simulink model "acvh_controller_mark1"  (R2020b)
settings: Solver=FixedStepAuto  StartTime=0.0  StopTime=Inf  RelTol=1e-3  EnableMultiTasking=on
values from neighbouring files (symbols this model uses):
  D = .2540    (= 0.254)    [iris_quadcopter_specs.m]
  SampleTime = 0.001    [iris_quadcopter_specs.m]
undefined symbols (not defined in the file or in its folder): dev, DiscIntNeverNeededParam, Main, pwm_output0
libraries: pid_lib x6, px4uORBlib x5, sharedtransform x1, px4lib x1
settings Model: SimulationMode=external  ExtModeTrigDuration=10  Creator=sid  LastModifiedBy=sid
settings SolverCC: PositivePriorityOrder=on
settings OptimizationCC: EnhancedBackFolding=on  PassReuseOutputArgsAs=Individual arguments  ZeroExternalMemoryAtStartup=off  ZeroInternalMemoryAtStartup=off  MaxStackSize=64  OptimizeBlockOrder=speed  DifferentSizesBufferReuse=on  OptimizationCustomize=off  EfficientTunableParamExpr=on
settings DebuggingCC: ParameterTunabilityLossMsg=error
settings HardwareCC: ProdBitPerPointer=32  ProdBitPerSizeT=32  ProdBitPerPtrDiffT=32  ProdLargestAtomicInteger=Long  ProdLargestAtomicFloat=Double  ProdWordSize=32  ProdLongLongMode=on  ProdHWDeviceType=ARM Compatible->ARM Cortex
settings SFSimCC: MATLABDynamicMemAlloc=off  SimTargetLang=C++
settings RTWCC: Description=Embedded Coder  SystemTargetFile=ert.tlc  HardwareBoard=PX4 Host Target  TLCOptions="-aInlineSetEventsForThisBaseRateFcn=TLC_FALSE -aSuppressMultiTaskScheduler=TLC_FALSE  -aRateBasedStepFcn=0"  TemplateMakefile=ert_default_tmf  Toolchain=GNU Tools for PX4 Autopilots  PortableWordSizes=on  TargetLang=C++
settings CodeAppCC: ForceParamTrailComments=on  IgnoreCustomStorageClasses=off  OperatorAnnotations=on  SimulinkDataObjDesc=on  SFDataObjDesc=on  InsertBlockDesc=on
settings ERTTargetCC: ExtMode=on  ExtModeMexArgs='127.0.0.1' 1 17725

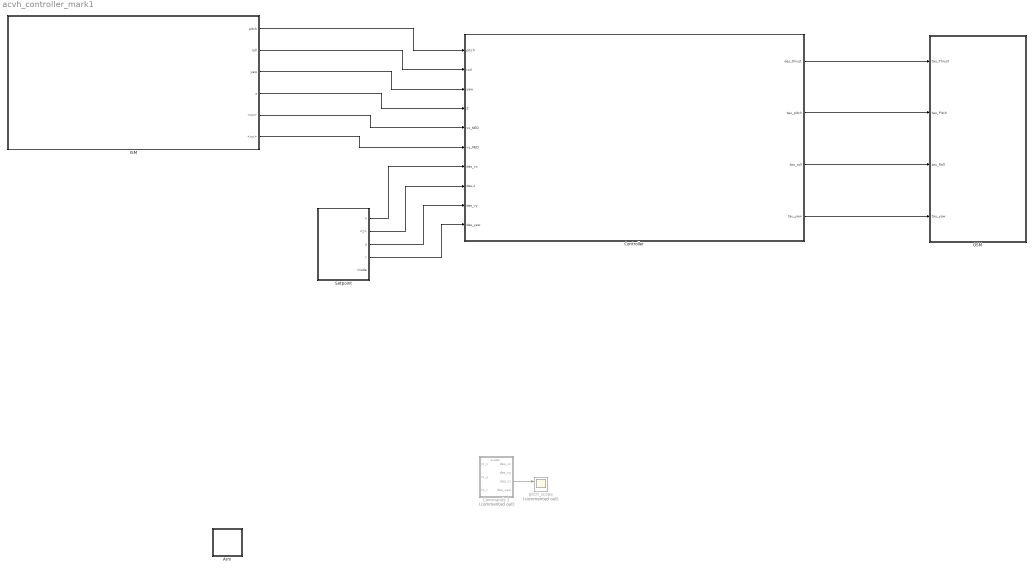
== system acvh_controller_mark1 ==
  Arm : Subsystem
  Commands 1 : Subsystem  Commented=on
  Controller : Subsystem
  ISM : Subsystem
  OSM : Subsystem
  Setpoint : Subsystem
  pitch_scope : Scope  Commented=on  NumInputPorts=2
  wires:
  Controller/1(des_thrust) -> OSM/1(tau_Thrust)
  Controller/3(tau_roll) -> OSM/3(tau_Roll)
  Controller/4(tau_yaw) -> OSM/4(tau_yaw)
  Commands 1/3(des_vz) -> pitch_scope/1
  Controller/2(tau_pitch) -> OSM/2(tau_Pitch)
  ISM/1(pitch) -> Controller/1(pitch)
  ISM/2(roll) -> Controller/2(roll)
  ISM/3(yaw) -> Controller/3(yaw)
  ISM/4(z) -> Controller/4(Z)
  ISM/5(<vx>) -> Controller/5(vx_NED)
  ISM/6(<vy>) -> Controller/6(vy_NED)
  Setpoint/4(r) -> Controller/10(des_yaw)
  Setpoint/1(x) -> Controller/7(des_vx)
  Setpoint/3(y) -> Controller/9(des_vy)
  Setpoint/2(<z>) -> Controller/8(des-z)

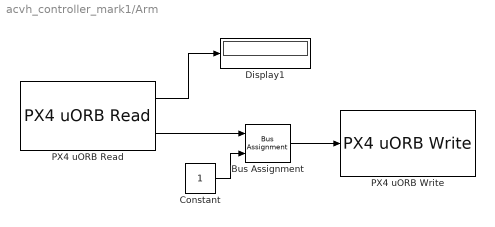
== system acvh_controller_mark1/Arm ==
  Bus Assignment : BusAssignment  AssignedSignals=armed
  Constant : Constant  OutDataTypeStr=Inherit: Inherit via back propagation  SampleTime=SampleTime
  Display1 : Display
  PX4 uORB Read : px4uORBlib/PX4 uORB Read  uORBTopic=actuator_armed  selectInstance=actuator_armed  SampleTime=SampleTime  BlockingMode=off  BlockTimeout=1e-3
      settings: SourceProductBaseCode=PX4AUTOPILOTS
  PX4 uORB Write : px4uORBlib/PX4 uORB Write  uORBTopic=actuator_armed  selectInstance=actuator_armed  MessageQueueLen=1
      settings: SourceProductBaseCode=PX4AUTOPILOTS
  wires:
  PX4 uORB Read/2 -> Bus Assignment/1
  PX4 uORB Read/1 -> Display1/1
  Bus Assignment/1 -> PX4 uORB Write/1
  Constant/1 -> Bus Assignment/2

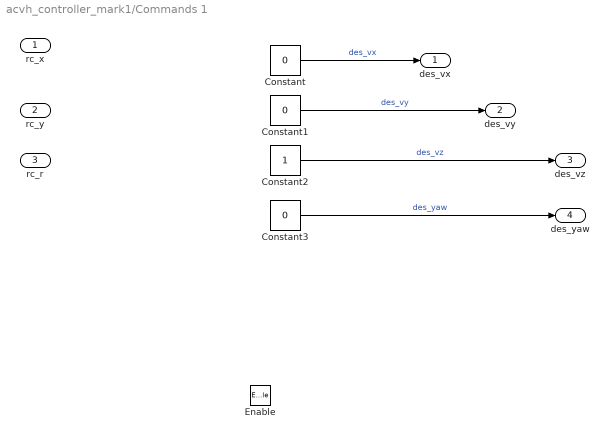
== system acvh_controller_mark1/Commands 1 ==
  rc_x : Inport
  rc_y : Inport  Port=2
  rc_r : Inport  Port=3
  Enable : EnablePort
  Constant : Constant  Value=0
  Constant1 : Constant  Value=0
  Constant2 : Constant
  Constant3 : Constant  Value=0
  des_vx : Outport
  des_vy : Outport  Port=2
  des_vz : Outport  Port=3
  des_yaw : Outport  Port=4
  wires:
  Constant1/1 -> des_vy/1  "des_vy"
  Constant/1 -> des_vx/1  "des_vx"
  Constant2/1 -> des_vz/1  "des_vz"
  Constant3/1 -> des_yaw/1  "des_yaw"

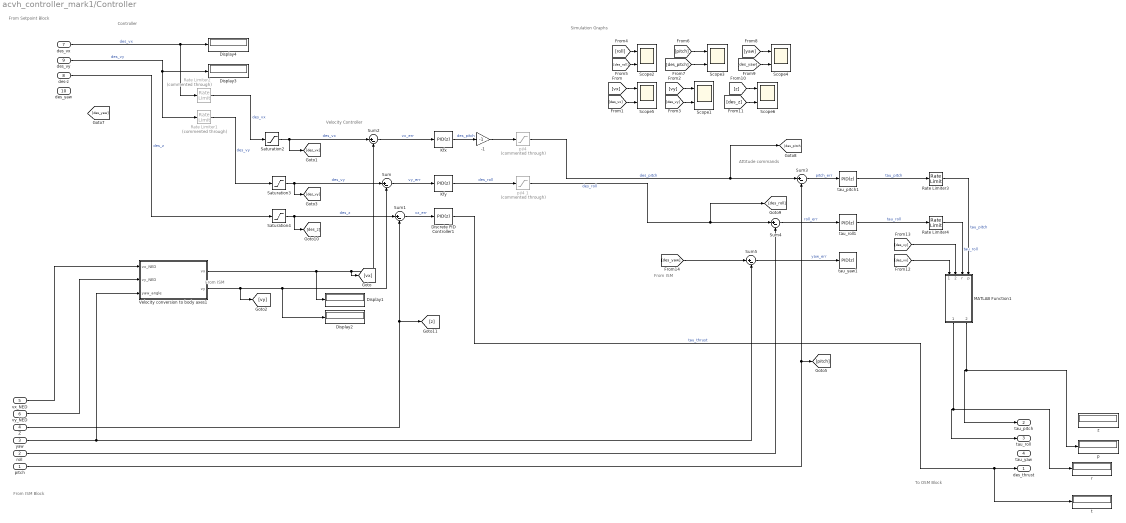
== system acvh_controller_mark1/Controller ==
  note: Simulation Graphs
  note: From Setpoint Block
  note: From ISM
  note: From ISM
  note: Controller
  note: Attitude commands
  note: Velocity Controller
  note: From ISM Block
  note: To OSM Block
  pitch : Inport
  roll : Inport  Port=2
  yaw : Inport  Port=3
  Z : Inport  Port=4
  vx_NED : Inport  Port=5
  vy_NED : Inport  Port=6
  des_vx : Inport  Port=7
  des-z : Inport  Port=8
  des_vy : Inport  Port=9
  des_yaw : Inport  Port=10
  -1 : Gain  Gain=-1
  Discrete PID Controller1 : pid_lib/PID Controller  Controller=PID  Form=Parallel  TimeDomain=Discrete-time  UseExternalTs=off  SampleTime=SampleTime  IntegratorMethod=Trapezoidal  FilterMethod=Trapezoidal  ControllerParametersSource=internal  P=-0.0534535340221691  I=-0.00566953766767209  D=-0.123220888476467  UseFilter=on  N=26.3491959083223  TunerSelectOption=Transfer Function Based (PID Tuner App)  InitialConditionSource=internal  InitialConditionForIntegrator=0  InitialConditionForFilter=0  DifferentiatorICPrevScaledInput=0  ExternalReset=none  TrackingMode=off  Kt=1  LimitOutput=off  SatLimitsSource=internal  UpperSaturationLimit=10  LowerSaturationLimit=-.05  LinearizeAsGain=off  AntiWindupMode=back-calculation  Kb=10  POutMin=[]  POutMax=[]  IOutMin=[]  IOutMax=[]  DOutMin=[]  DOutMax=[]  NOutMin=[]  NOutMax=[]  SumOutMin=[]  SumOutMax=[]  SaturationOutMin=[]  SaturationOutMax=[]  PParamMin=[]  PParamMax=[]  IParamMin=[]  IParamMax=[]  DParamMin=[]  DParamMax=[]  NParamMin=[]  NParamMax=[]  KbParamMin=[]  KbParamMax=[]  KtParamMin=[]  KtParamMax=[]  KbOutMin=[]  KbOutMax=[]  KtOutMin=[]  KtOutMax=[]  IntegratorOutMin=[]  IntegratorOutMax=[]  FilterOutMin=[]  FilterOutMax=[]  SumI1OutMin=[]  SumI1OutMax=[]  SumI2OutMin=[]  SumI2OutMax=[]  SumI3OutMin=[]  SumI3OutMax=[]  SumI4OutMin=[]  SumI4OutMax=[]  SumDOutMin=[]  SumDOutMax=[]  DifferentiatorOutMin=[]  DifferentiatorOutMax=[]  FilterDiffOutCoefMin=[]  FilterDiffOutCoefMax=[]  ReciprocalOutMin=[]  ReciprocalOutMax=[]  SumDenOutMin=[]  SumDenOutMax=[]  SumNumOutMin=[]  SumNumOutMax=[]  DivideOutMin=[]  DivideOutMax=[]  UdiffTsProdOutMin=[]  UdiffTsProdOutMax=[]  NTsProdOutMin=[]  NTsProdOutMax=[]  UintegralTsProdOutMin=[]  UintegralTsProdOutMax=[]  UngainTsProdOutMin=[]  UngainTsProdOutMax=[]  IntegratorContinuousStateAttributes=''  IntegratorStateMustResolveToSignalObject=off  IntegratorRTWStateStorageClass=Auto  FilterContinuousStateAttributes=''  FilterStateMustResolveToSignalObject=off  FilterRTWStateStorageClass=Auto  ParallelPVariant=InternalParameters  IdealPVariant=Disabled  IVariant=InternalParameters  DVariant=InternalParameters  IntegratorVariant=Discrete  SatVariant=Disabled  AWVariant=Passthrough  PCopyVariant=Disabled  TRVariant=Disabled  FdbkBlocksVariant=Forward  IdealPFdbkVariant=Disabled  SatFdbkVariant=Disabled  DerivativeFilterVariant=TrapezoidalFilter  NVariant=InternalParameters  NCopyVariant=InternalParameters  FilterICVariant=InternalICsFilter  IntegratorICVariant=InternalICs  ExternalResetVariant=Disabled  TRSumVariant=Passthrough  SumFdbkVariant=Disabled  SumVariant=Sum_PID  TsampFilterVariant=InternalTs  TsampNgainVariant=Passthrough  TsampIntegralVariant=Passthrough  ExternalSaturationOutDataTypeStr=Inherit: Same as second input
  Display{1..4} (4 alike) : Display
  Kfx : pid_lib/PID Controller  Controller=PID  Form=Parallel  TimeDomain=Discrete-time  UseExternalTs=off  SampleTime=SampleTime  IntegratorMethod=Forward Euler  FilterMethod=Forward Euler  ControllerParametersSource=internal  P=0.183358617742533  I=0.0739424315877928  D=-0.024031657470412  UseFilter=on  N=7.50922781087257  TunerSelectOption=Transfer Function Based (PID Tuner App)  InitialConditionSource=internal  InitialConditionForIntegrator=0  InitialConditionForFilter=0  DifferentiatorICPrevScaledInput=0  ExternalReset=none  TrackingMode=off  Kt=1  LimitOutput=on  SatLimitsSource=internal  UpperSaturationLimit=pi/8  LowerSaturationLimit=-pi/8  LinearizeAsGain=off  AntiWindupMode=clamping  Kb=1  POutMin=[]  POutMax=[]  IOutMin=[]  IOutMax=[]  DOutMin=[]  DOutMax=[]  NOutMin=[]  NOutMax=[]  SumOutMin=[]  SumOutMax=[]  SaturationOutMin=[]  SaturationOutMax=[]  PParamMin=[]  PParamMax=[]  IParamMin=[]  IParamMax=[]  DParamMin=[]  DParamMax=[]  NParamMin=[]  NParamMax=[]  KbParamMin=[]  KbParamMax=[]  KtParamMin=[]  KtParamMax=[]  KbOutMin=[]  KbOutMax=[]  KtOutMin=[]  KtOutMax=[]  IntegratorOutMin=[]  IntegratorOutMax=[]  FilterOutMin=[]  FilterOutMax=[]  SumI1OutMin=[]  SumI1OutMax=[]  SumI2OutMin=[]  SumI2OutMax=[]  SumI3OutMin=[]  SumI3OutMax=[]  SumI4OutMin=[]  SumI4OutMax=[]  SumDOutMin=[]  SumDOutMax=[]  DifferentiatorOutMin=[]  DifferentiatorOutMax=[]  FilterDiffOutCoefMin=[]  FilterDiffOutCoefMax=[]  ReciprocalOutMin=[]  ReciprocalOutMax=[]  SumDenOutMin=[]  SumDenOutMax=[]  SumNumOutMin=[]  SumNumOutMax=[]  DivideOutMin=[]  DivideOutMax=[]  UdiffTsProdOutMin=[]  UdiffTsProdOutMax=[]  NTsProdOutMin=[]  NTsProdOutMax=[]  UintegralTsProdOutMin=[]  UintegralTsProdOutMax=[]  UngainTsProdOutMin=[]  UngainTsProdOutMax=[]  IntegratorContinuousStateAttributes=''  IntegratorStateMustResolveToSignalObject=off  IntegratorRTWStateStorageClass=Auto  FilterContinuousStateAttributes=''  FilterStateMustResolveToSignalObject=off  FilterRTWStateStorageClass=Auto  ParallelPVariant=InternalParameters  IdealPVariant=Disabled  IVariant=InternalParameters  DVariant=InternalParameters  IntegratorVariant=Discrete  SatVariant=Enabled  AWVariant=DiscClampingParallel  PCopyVariant=Disabled  TRVariant=Disabled  FdbkBlocksVariant=Forward  IdealPFdbkVariant=Disabled  SatFdbkVariant=Disabled  DerivativeFilterVariant=ForwardEulerFilter  NVariant=InternalParameters  NCopyVariant=Disabled  FilterICVariant=InternalICsFilter  IntegratorICVariant=InternalICs  ExternalResetVariant=Disabled  TRSumVariant=Passthrough  SumFdbkVariant=Disabled  SumVariant=Sum_PID  TsampFilterVariant=InternalTs  TsampNgainVariant=Passthrough  TsampIntegralVariant=Passthrough  ExternalSaturationOutDataTypeStr=Inherit: Same as second input
  Kfy : pid_lib/PID Controller  Controller=PID  Form=Parallel  TimeDomain=Discrete-time  UseExternalTs=off  SampleTime=SampleTime  IntegratorMethod=Forward Euler  FilterMethod=Forward Euler  ControllerParametersSource=internal  P=0.183358617742446  I=0.0739424315877666  D=-0.0240316574704006  UseFilter=on  N=7.50922781087257  TunerSelectOption=Transfer Function Based (PID Tuner App)  InitialConditionSource=internal  InitialConditionForIntegrator=0  InitialConditionForFilter=0  DifferentiatorICPrevScaledInput=0  ExternalReset=none  TrackingMode=off  Kt=1  LimitOutput=on  SatLimitsSource=internal  UpperSaturationLimit=pi/8  LowerSaturationLimit=-pi/8  LinearizeAsGain=off  AntiWindupMode=clamping  Kb=1  POutMin=[]  POutMax=[]  IOutMin=[]  IOutMax=[]  DOutMin=[]  DOutMax=[]  NOutMin=[]  NOutMax=[]  SumOutMin=[]  SumOutMax=[]  SaturationOutMin=[]  SaturationOutMax=[]  PParamMin=[]  PParamMax=[]  IParamMin=[]  IParamMax=[]  DParamMin=[]  DParamMax=[]  NParamMin=[]  NParamMax=[]  KbParamMin=[]  KbParamMax=[]  KtParamMin=[]  KtParamMax=[]  KbOutMin=[]  KbOutMax=[]  KtOutMin=[]  KtOutMax=[]  IntegratorOutMin=[]  IntegratorOutMax=[]  FilterOutMin=[]  FilterOutMax=[]  SumI1OutMin=[]  SumI1OutMax=[]  SumI2OutMin=[]  SumI2OutMax=[]  SumI3OutMin=[]  SumI3OutMax=[]  SumI4OutMin=[]  SumI4OutMax=[]  SumDOutMin=[]  SumDOutMax=[]  DifferentiatorOutMin=[]  DifferentiatorOutMax=[]  FilterDiffOutCoefMin=[]  FilterDiffOutCoefMax=[]  ReciprocalOutMin=[]  ReciprocalOutMax=[]  SumDenOutMin=[]  SumDenOutMax=[]  SumNumOutMin=[]  SumNumOutMax=[]  DivideOutMin=[]  DivideOutMax=[]  UdiffTsProdOutMin=[]  UdiffTsProdOutMax=[]  NTsProdOutMin=[]  NTsProdOutMax=[]  UintegralTsProdOutMin=[]  UintegralTsProdOutMax=[]  UngainTsProdOutMin=[]  UngainTsProdOutMax=[]  IntegratorContinuousStateAttributes=''  IntegratorStateMustResolveToSignalObject=off  IntegratorRTWStateStorageClass=Auto  FilterContinuousStateAttributes=''  FilterStateMustResolveToSignalObject=off  FilterRTWStateStorageClass=Auto  ParallelPVariant=InternalParameters  IdealPVariant=Disabled  IVariant=InternalParameters  DVariant=InternalParameters  IntegratorVariant=Discrete  SatVariant=Enabled  AWVariant=DiscClampingParallel  PCopyVariant=Disabled  TRVariant=Disabled  FdbkBlocksVariant=Forward  IdealPFdbkVariant=Disabled  SatFdbkVariant=Disabled  DerivativeFilterVariant=ForwardEulerFilter  NVariant=InternalParameters  NCopyVariant=Disabled  FilterICVariant=InternalICsFilter  IntegratorICVariant=InternalICs  ExternalResetVariant=Disabled  TRSumVariant=Passthrough  SumFdbkVariant=Disabled  SumVariant=Sum_PID  TsampFilterVariant=InternalTs  TsampNgainVariant=Passthrough  TsampIntegralVariant=Passthrough  ExternalSaturationOutDataTypeStr=Inherit: Same as second input
  MATLAB Function1 : MATLAB Function  TreatAsAtomicUnit=on
  Rate Limiter1 : RateLimiter  Commented=through  RisingSlewLimit=3  FallingSlewLimit=-3
  Rate Limiter2 : RateLimiter  Commented=through  RisingSlewLimit=3  FallingSlewLimit=-3
  Rate Limiter3 : RateLimiter  RisingSlewLimit=.001  FallingSlewLimit=-.001  SampleTimeMode=inherited
  Rate Limiter4 : RateLimiter  RisingSlewLimit=.001  FallingSlewLimit=-.001  SampleTimeMode=inherited
  Saturation2 : Saturate  UpperLimit=8  LowerLimit=-8  LinearizeAsGain=off
  Saturation3 : Saturate  UpperLimit=8  LowerLimit=-8  LinearizeAsGain=off
  Saturation4 : Saturate  UpperLimit=0  LowerLimit=-6
  Scope{1..6} (6 alike) : Scope  NumInputPorts=2
  Sum{,1..5} (6 alike) : Sum  Inputs=|+-
  Velocity conversion to body axes1 : Subsystem
  p : Display
  pi/4 : Saturate  Commented=through  UpperLimit=pi/16  LowerLimit=-pi/16
  pi/4 1 : Saturate  Commented=through  UpperLimit=pi/16  LowerLimit=-pi/16
  r : Display
  t : Display
  tau_pitch1 : pid_lib/PID Controller  Controller=PID  Form=Parallel  TimeDomain=Discrete-time  UseExternalTs=off  SampleTime=SampleTime  IntegratorMethod=Forward Euler  FilterMethod=Forward Euler  ControllerParametersSource=internal  P=0.0543673511512337  I=0.0109980209644375  D=0.0263229670839572  UseFilter=on  N=347.83750102845  TunerSelectOption=Transfer Function Based (PID Tuner App)  InitialConditionSource=internal  InitialConditionForIntegrator=0  InitialConditionForFilter=0  DifferentiatorICPrevScaledInput=0  ExternalReset=none  TrackingMode=off  Kt=1  LimitOutput=on  SatLimitsSource=internal  UpperSaturationLimit=.0005  LowerSaturationLimit=-.0005  LinearizeAsGain=off  AntiWindupMode=none  Kb=1  POutMin=[]  POutMax=[]  IOutMin=[]  IOutMax=[]  DOutMin=[]  DOutMax=[]  NOutMin=[]  NOutMax=[]  SumOutMin=[]  SumOutMax=[]  SaturationOutMin=[]  SaturationOutMax=[]  PParamMin=[]  PParamMax=[]  IParamMin=[]  IParamMax=[]  DParamMin=[]  DParamMax=[]  NParamMin=[]  NParamMax=[]  KbParamMin=[]  KbParamMax=[]  KtParamMin=[]  KtParamMax=[]  KbOutMin=[]  KbOutMax=[]  KtOutMin=[]  KtOutMax=[]  IntegratorOutMin=[]  IntegratorOutMax=[]  FilterOutMin=[]  FilterOutMax=[]  SumI1OutMin=[]  SumI1OutMax=[]  SumI2OutMin=[]  SumI2OutMax=[]  SumI3OutMin=[]  SumI3OutMax=[]  SumI4OutMin=[]  SumI4OutMax=[]  SumDOutMin=[]  SumDOutMax=[]  DifferentiatorOutMin=[]  DifferentiatorOutMax=[]  FilterDiffOutCoefMin=[]  FilterDiffOutCoefMax=[]  ReciprocalOutMin=[]  ReciprocalOutMax=[]  SumDenOutMin=[]  SumDenOutMax=[]  SumNumOutMin=[]  SumNumOutMax=[]  DivideOutMin=[]  DivideOutMax=[]  UdiffTsProdOutMin=[]  UdiffTsProdOutMax=[]  NTsProdOutMin=[]  NTsProdOutMax=[]  UintegralTsProdOutMin=[]  UintegralTsProdOutMax=[]  UngainTsProdOutMin=[]  UngainTsProdOutMax=[]  IntegratorContinuousStateAttributes=''  IntegratorStateMustResolveToSignalObject=off  IntegratorRTWStateStorageClass=Auto  FilterContinuousStateAttributes=''  FilterStateMustResolveToSignalObject=off  FilterRTWStateStorageClass=Auto  ParallelPVariant=InternalParameters  IdealPVariant=Disabled  IVariant=InternalParameters  DVariant=InternalParameters  IntegratorVariant=Discrete  SatVariant=Enabled  AWVariant=Passthrough  PCopyVariant=Disabled  TRVariant=Disabled  FdbkBlocksVariant=Forward  IdealPFdbkVariant=Disabled  SatFdbkVariant=Disabled  DerivativeFilterVariant=ForwardEulerFilter  NVariant=InternalParameters  NCopyVariant=Disabled  FilterICVariant=InternalICsFilter  IntegratorICVariant=InternalICs  ExternalResetVariant=Disabled  TRSumVariant=Passthrough  SumFdbkVariant=Disabled  SumVariant=Sum_PID  TsampFilterVariant=InternalTs  TsampNgainVariant=Passthrough  TsampIntegralVariant=Passthrough  ExternalSaturationOutDataTypeStr=Inherit: Same as second input
  tau_roll1 : pid_lib/PID Controller  Controller=PID  Form=Parallel  TimeDomain=Discrete-time  UseExternalTs=off  SampleTime=SampleTime  IntegratorMethod=Forward Euler  FilterMethod=Forward Euler  ControllerParametersSource=internal  P=-0.0543673511512337  I=-0.0109980209644375  D=-0.0263229670839572  UseFilter=on  N=347.83750102845  TunerSelectOption=Transfer Function Based (PID Tuner App)  InitialConditionSource=internal  InitialConditionForIntegrator=0  InitialConditionForFilter=0  DifferentiatorICPrevScaledInput=0  ExternalReset=none  TrackingMode=off  Kt=1  LimitOutput=on  SatLimitsSource=internal  UpperSaturationLimit=.0005  LowerSaturationLimit=-.0005  LinearizeAsGain=off  AntiWindupMode=none  Kb=1  POutMin=[]  POutMax=[]  IOutMin=[]  IOutMax=[]  DOutMin=[]  DOutMax=[]  NOutMin=[]  NOutMax=[]  SumOutMin=[]  SumOutMax=[]  SaturationOutMin=[]  SaturationOutMax=[]  PParamMin=[]  PParamMax=[]  IParamMin=[]  IParamMax=[]  DParamMin=[]  DParamMax=[]  NParamMin=[]  NParamMax=[]  KbParamMin=[]  KbParamMax=[]  KtParamMin=[]  KtParamMax=[]  KbOutMin=[]  KbOutMax=[]  KtOutMin=[]  KtOutMax=[]  IntegratorOutMin=[]  IntegratorOutMax=[]  FilterOutMin=[]  FilterOutMax=[]  SumI1OutMin=[]  SumI1OutMax=[]  SumI2OutMin=[]  SumI2OutMax=[]  SumI3OutMin=[]  SumI3OutMax=[]  SumI4OutMin=[]  SumI4OutMax=[]  SumDOutMin=[]  SumDOutMax=[]  DifferentiatorOutMin=[]  DifferentiatorOutMax=[]  FilterDiffOutCoefMin=[]  FilterDiffOutCoefMax=[]  ReciprocalOutMin=[]  ReciprocalOutMax=[]  SumDenOutMin=[]  SumDenOutMax=[]  SumNumOutMin=[]  SumNumOutMax=[]  DivideOutMin=[]  DivideOutMax=[]  UdiffTsProdOutMin=[]  UdiffTsProdOutMax=[]  NTsProdOutMin=[]  NTsProdOutMax=[]  UintegralTsProdOutMin=[]  UintegralTsProdOutMax=[]  UngainTsProdOutMin=[]  UngainTsProdOutMax=[]  IntegratorContinuousStateAttributes=''  IntegratorStateMustResolveToSignalObject=off  IntegratorRTWStateStorageClass=Auto  FilterContinuousStateAttributes=''  FilterStateMustResolveToSignalObject=off  FilterRTWStateStorageClass=Auto  ParallelPVariant=InternalParameters  IdealPVariant=Disabled  IVariant=InternalParameters  DVariant=InternalParameters  IntegratorVariant=Discrete  SatVariant=Enabled  AWVariant=Passthrough  PCopyVariant=Disabled  TRVariant=Disabled  FdbkBlocksVariant=Forward  IdealPFdbkVariant=Disabled  SatFdbkVariant=Disabled  DerivativeFilterVariant=ForwardEulerFilter  NVariant=InternalParameters  NCopyVariant=Disabled  FilterICVariant=InternalICsFilter  IntegratorICVariant=InternalICs  ExternalResetVariant=Disabled  TRSumVariant=Passthrough  SumFdbkVariant=Disabled  SumVariant=Sum_PID  TsampFilterVariant=InternalTs  TsampNgainVariant=Passthrough  TsampIntegralVariant=Passthrough  ExternalSaturationOutDataTypeStr=Inherit: Same as second input
  tau_yaw1 : pid_lib/PID Controller  Controller=PID  Form=Parallel  TimeDomain=Discrete-time  UseExternalTs=off  SampleTime=SampleTime  IntegratorMethod=Forward Euler  FilterMethod=Forward Euler  ControllerParametersSource=internal  P=-0.564155915391973  I=-0.130215223566003  D=-0.447814603729917  UseFilter=on  N=347.83750102845  TunerSelectOption=Transfer Function Based (PID Tuner App)  InitialConditionSource=internal  InitialConditionForIntegrator=0  InitialConditionForFilter=0  DifferentiatorICPrevScaledInput=0  ExternalReset=none  TrackingMode=off  Kt=1  LimitOutput=on  SatLimitsSource=internal  UpperSaturationLimit=0.1  LowerSaturationLimit=-0.1  LinearizeAsGain=off  AntiWindupMode=none  Kb=1  POutMin=[]  POutMax=[]  IOutMin=[]  IOutMax=[]  DOutMin=[]  DOutMax=[]  NOutMin=[]  NOutMax=[]  SumOutMin=[]  SumOutMax=[]  SaturationOutMin=[]  SaturationOutMax=[]  PParamMin=[]  PParamMax=[]  IParamMin=[]  IParamMax=[]  DParamMin=[]  DParamMax=[]  NParamMin=[]  NParamMax=[]  KbParamMin=[]  KbParamMax=[]  KtParamMin=[]  KtParamMax=[]  KbOutMin=[]  KbOutMax=[]  KtOutMin=[]  KtOutMax=[]  IntegratorOutMin=[]  IntegratorOutMax=[]  FilterOutMin=[]  FilterOutMax=[]  SumI1OutMin=[]  SumI1OutMax=[]  SumI2OutMin=[]  SumI2OutMax=[]  SumI3OutMin=[]  SumI3OutMax=[]  SumI4OutMin=[]  SumI4OutMax=[]  SumDOutMin=[]  SumDOutMax=[]  DifferentiatorOutMin=[]  DifferentiatorOutMax=[]  FilterDiffOutCoefMin=[]  FilterDiffOutCoefMax=[]  ReciprocalOutMin=[]  ReciprocalOutMax=[]  SumDenOutMin=[]  SumDenOutMax=[]  SumNumOutMin=[]  SumNumOutMax=[]  DivideOutMin=[]  DivideOutMax=[]  UdiffTsProdOutMin=[]  UdiffTsProdOutMax=[]  NTsProdOutMin=[]  NTsProdOutMax=[]  UintegralTsProdOutMin=[]  UintegralTsProdOutMax=[]  UngainTsProdOutMin=[]  UngainTsProdOutMax=[]  IntegratorContinuousStateAttributes=''  IntegratorStateMustResolveToSignalObject=off  IntegratorRTWStateStorageClass=Auto  FilterContinuousStateAttributes=''  FilterStateMustResolveToSignalObject=off  FilterRTWStateStorageClass=Auto  ParallelPVariant=InternalParameters  IdealPVariant=Disabled  IVariant=InternalParameters  DVariant=InternalParameters  IntegratorVariant=Discrete  SatVariant=Enabled  AWVariant=Passthrough  PCopyVariant=Disabled  TRVariant=Disabled  FdbkBlocksVariant=Forward  IdealPFdbkVariant=Disabled  SatFdbkVariant=Disabled  DerivativeFilterVariant=ForwardEulerFilter  NVariant=InternalParameters  NCopyVariant=Disabled  FilterICVariant=InternalICsFilter  IntegratorICVariant=InternalICs  ExternalResetVariant=Disabled  TRSumVariant=Passthrough  SumFdbkVariant=Disabled  SumVariant=Sum_PID  TsampFilterVariant=InternalTs  TsampNgainVariant=Passthrough  TsampIntegralVariant=Passthrough  ExternalSaturationOutDataTypeStr=Inherit: Same as second input
  z : Display
  des_thrust : Outport
  tau_pitch : Outport  Port=2
  tau_roll : Outport  Port=3
  tau_yaw : Outport  Port=4
  wires:
  Sum/1 -> Kfy/1  "vy_err"
  [des_vy] -> Scope1/2
  [pitch] -> Scope3/1
  -1/1 -> pi/4/1
  [yaw] -> Scope4/1
  Kfx/1 -> -1/1  "des_pitch"
  Velocity conversion to body axes1/1(vx) -> Display1/1, Sum2/2, [vx]
  roll/1 -> Sum4/2
  vy_NED/1 -> Velocity conversion to body axes1/2(vy_NED)
  Sum1/1 -> Discrete PID Controller1/1  "vz_err"
  [des_z] -> Scope6/2
  pitch/1 -> [pitch], Sum3/2
  Velocity conversion to body axes1/2(vy) -> Display2/1, Sum/2, [vy]
  Rate Limiter2/1 -> Saturation2/1  "des_vx"
  vx_NED/1 -> Velocity conversion to body axes1/1(vx_NED)
  pi/4 1/1 -> [des_roll], Sum4/1  "des_roll"
  Rate Limiter1/1 -> Saturation3/1  "des_vy"
  Kfy/1 -> pi/4 1/1  "des_roll"
  Sum4/1 -> tau_roll1/1  "roll_err"
  [des_roll] -> Scope2/2
  [des_pitch] -> Scope3/2
  [des_yaw] -> Scope4/2
  Z/1 -> Sum1/2, [z]
  Sum2/1 -> Kfx/1  "vx_err"
  [vx] -> Scope5/1
  pi/4/1 -> [des_pitch], Sum3/1  "des_pitch"
  [z] -> Scope6/1
  Saturation2/1 -> Sum2/1, [des_vx]  "des_vx"
  [roll] -> Scope2/1
  [vy] -> Scope1/1
  [des_vx] -> Scope5/2
  Sum3/1 -> tau_pitch1/1  "pitch_err"
  Sum5/1 -> tau_yaw1/1  "yaw_err"
  Saturation4/1 -> [des_z], Sum1/1  "des_z"
  Discrete PID Controller1/1 -> t/1, des_thrust/1  "tau_thrust"
  yaw/1 -> Sum5/2, Velocity conversion to body axes1/3(yaw_angle)
  des-z/1 -> Saturation4/1  "des_z"
  des_vx/1 -> Rate Limiter2/1, Display4/1  "des_vx"
  des_vy/1 -> Rate Limiter1/1, Display3/1  "des_vy"
  [des_vx] -> MATLAB Function1/1(des_vx)
  MATLAB Function1/2(tau_pitch) -> tau_pitch/1, p/1
  MATLAB Function1/1(tau_roll) -> tau_roll/1, r/1
  tau_roll1/1 -> Rate Limiter4/1  "tau_roll"
  tau_pitch1/1 -> Rate Limiter3/1  "tau_pitch"
  Rate Limiter4/1 -> MATLAB Function1/3(r)  "tau_roll"
  Rate Limiter3/1 -> MATLAB Function1/4(p)  "tau_pitch"
  [des_vy] -> MATLAB Function1/2(des_vy)
  [des_yaw] -> Sum5/1
  Saturation3/1 -> Sum/1, [des_vy]  "des_vy"

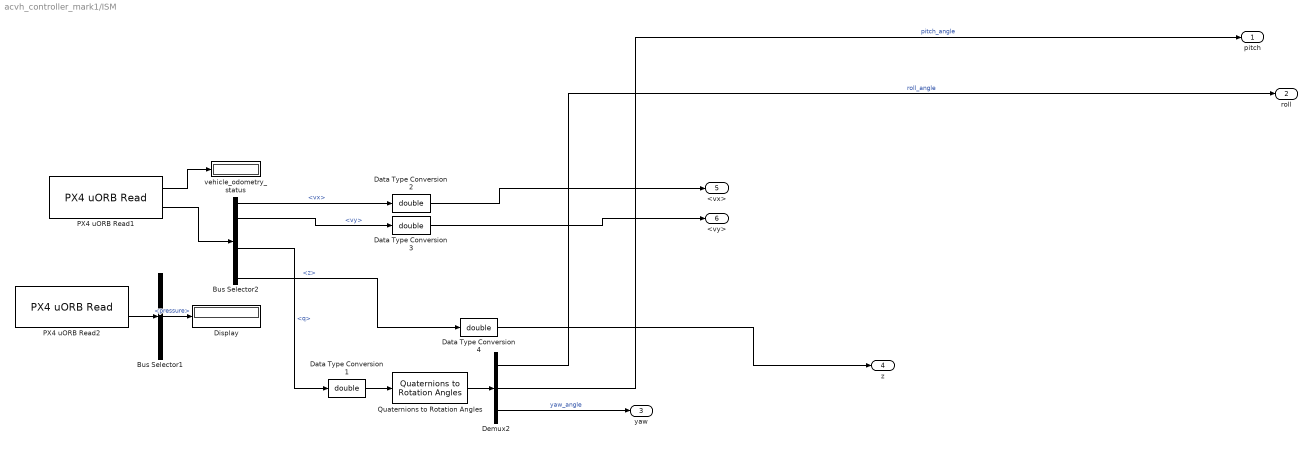
== system acvh_controller_mark1/ISM ==
  Bus Selector1 : BusSelector  OutputSignals=pressure
  Bus Selector2 : BusSelector  OutputSignals=vx,vy,vz,q,yawspeed,z
  Data Type Conversion{1..4} (4 alike) : DataTypeConversion  OutDataTypeStr=double
  Demux2 : Demux  Outputs=3
  Display : Display
  PX4 uORB Read1 : px4uORBlib/PX4 uORB Read  uORBTopic=vehicle_odometry  selectInstance=vehicle_odometry  SampleTime=SampleTime  BlockingMode=off  BlockTimeout=1e-3
      settings: SourceProductBaseCode=PX4AUTOPILOTS
  PX4 uORB Read2 : px4uORBlib/PX4 uORB Read  uORBTopic=sensor_baro  selectInstance=sensor_baro  SampleTime=.001  BlockingMode=off  BlockTimeout=1e-3
      settings: SourceProductBaseCode=PX4AUTOPILOTS
  Quaternions to Rotation Angles : sharedtransform/Quaternions to Rotation Angles  rotationOrder=XYZ  aMode=aMode
      settings: SourceProductBaseCode=AE,PW,MT,UV,VE,VP
  vehicle_odometry_status : Display
  pitch : Outport
  roll : Outport  Port=2
  yaw : Outport  Port=3
  z : Outport  Port=4
  <vx> : Outport  Port=5
  <vy> : Outport  Port=6
  wires:
  PX4 uORB Read1/1 -> vehicle_odometry_status/1
  Bus Selector2/4 -> Data Type Conversion1/1  "<q>"
  PX4 uORB Read1/2 -> Bus Selector2/1
  Demux2/2 -> pitch/1  "pitch_angle"
  Demux2/3 -> yaw/1  "yaw_angle"
  Data Type Conversion1/1 -> Quaternions to Rotation Angles/1
  Quaternions to Rotation Angles/1 -> Demux2/1
  Demux2/1 -> roll/1  "roll_angle"
  PX4 uORB Read2/2 -> Bus Selector1/1
  Bus Selector1/1 -> Display/1  "<pressure>"
  Bus Selector2/1 -> Data Type Conversion2/1  "<vx>"
  Data Type Conversion2/1 -> <vx>/1
  Bus Selector2/2 -> Data Type Conversion3/1  "<vy>"
  Data Type Conversion3/1 -> <vy>/1
  Bus Selector2/6 -> Data Type Conversion4/1  "<z>"
  Data Type Conversion4/1 -> z/1

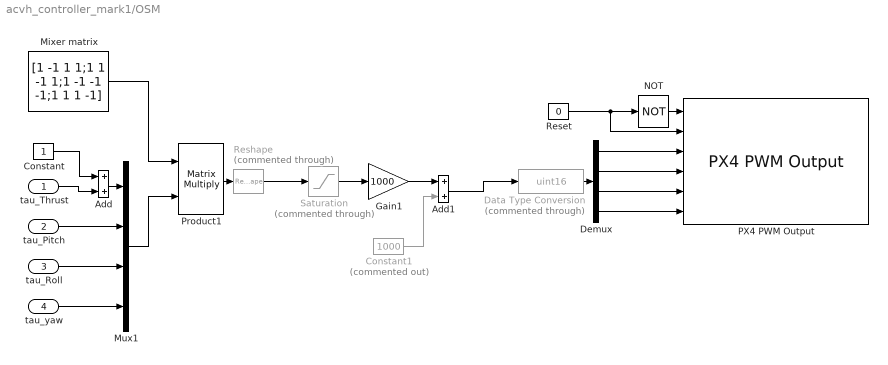
== system acvh_controller_mark1/OSM ==
  tau_Thrust : Inport
  tau_Pitch : Inport  Port=2
  tau_Roll : Inport  Port=3
  tau_yaw : Inport  Port=4
  Add : Sum
  Add1 : Sum
  Constant : Constant  SampleTime=SampleTime
  Constant1 : Constant  Commented=on  Value=1000  SampleTime=SampleTime
  Data Type Conversion : DataTypeConversion  Commented=through  OutDataTypeStr=uint16
  Demux : Demux
  Gain1 : Gain  Gain=1000  OutDataTypeStr=uint16
  Mixer matrix : Constant  Value=[1 -1 1 1;1 1 -1 1;1 -1 -1 -1;1 1 1 -1]  OutDataTypeStr=Inherit: Inherit via back propagation
  Mux1 : Mux
  NOT : Logic  Operator=NOT  IconShape=distinctive  AllPortsSameDT=off  OutDataTypeStr=boolean
  PX4 PWM Output : px4lib/PX4 PWM Output  pwmDevice=Main (/dev/pwm_output0)  pwmChannel1_=on  pwmChannel2_=on  pwmChannel3_=on  pwmChannel4_=on  pwmChannel5_=off  pwmChannel6_=off  pwmChannel7_=off  pwmChannel8_=off  forceTerminateFailsafe=off  outputErrorStatus=off
      settings: SourceProductBaseCode=PX4AUTOPILOTS
  Product1 : Product  Multiplication=Matrix(*)  RndMeth=Zero
  Reset : Constant  Value=0  OutDataTypeStr=boolean  SampleTime=SampleTime
  Reshape : Reshape  Commented=through  OutputDimensionality=Row vector (2-D)
  Saturation : Saturate  Commented=through  UpperLimit=1  LowerLimit=0
  wires:
  NOT/1 -> PX4 PWM Output/1
  Mixer matrix/1 -> Product1/1
  tau_yaw/1 -> Mux1/4
  tau_Pitch/1 -> Mux1/2
  tau_Roll/1 -> Mux1/3
  Reset/1 -> PX4 PWM Output/2, NOT/1
  Demux/3 -> PX4 PWM Output/5
  Demux/2 -> PX4 PWM Output/4
  Mux1/1 -> Product1/2
  Demux/4 -> PX4 PWM Output/6
  Demux/1 -> PX4 PWM Output/3
  tau_Thrust/1 -> Add/2
  Add/1 -> Mux1/1
  Constant/1 -> Add/1
  Saturation/1 -> Gain1/1
  Product1/1 -> Reshape/1
  Reshape/1 -> Saturation/1
  Gain1/1 -> Add1/1
  Constant1/1 -> Add1/2
  Add1/1 -> Data Type Conversion/1
  Data Type Conversion/1 -> Demux/1

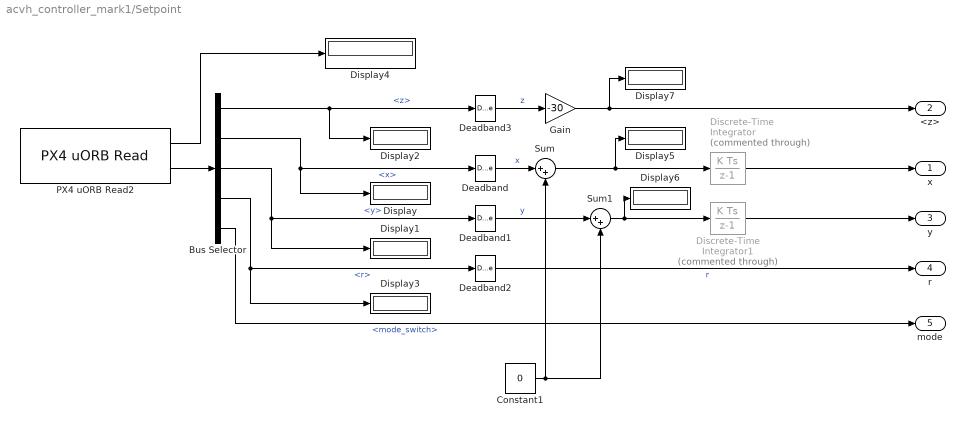
== system acvh_controller_mark1/Setpoint ==
  Bus Selector : BusSelector  OutputSignals=z,x,y,r,mode_switch
  Constant1 : Constant  Value=0  SampleTime=SampleTime
  Deadband{,1..3} (4 alike) : DeadZone  LowerValue=-0.05  UpperValue=0.05  SaturateOnIntegerOverflow=on
  Discrete-Time Integrator : DiscreteIntegrator  Commented=through  gainval=.001  SampleTime=SampleTime  ICPrevOutput=DiscIntNeverNeededParam  ICPrevScaledInput=DiscIntNeverNeededParam
  Discrete-Time Integrator1 : DiscreteIntegrator  Commented=through  gainval=.001  SampleTime=SampleTime  ICPrevOutput=DiscIntNeverNeededParam  ICPrevScaledInput=DiscIntNeverNeededParam
  Display{,1..7} (8 alike) : Display
  Gain : Gain  Gain=-30
  PX4 uORB Read2 : px4uORBlib/PX4 uORB Read  uORBTopic=manual_control_setpoint  selectInstance=manual_control_setpoint  SampleTime=SampleTime  BlockingMode=off  BlockTimeout=1e-3
      settings: SourceProductBaseCode=PX4AUTOPILOTS
  Sum : Sum  Inputs=|++
  Sum1 : Sum  Inputs=|++
  x : Outport
  <z> : Outport  Port=2
  y : Outport  Port=3
  r : Outport  Port=4
  mode : Outport  Port=5
  wires:
  Bus Selector/2 -> Display/1, Deadband/1  "<x>"
  Bus Selector/4 -> Display3/1, Deadband2/1  "<r>"
  Discrete-Time Integrator/1 -> x/1
  PX4 uORB Read2/1 -> Display4/1
  PX4 uORB Read2/2 -> Bus Selector/1
  Deadband/1 -> Sum/1  "x"
  Deadband2/1 -> r/1  "r"
  Bus Selector/1 -> Deadband3/1, Display2/1  "<z>"
  Deadband1/1 -> Sum1/1  "y"
  Constant1/1 -> Sum1/2, Sum/2
  Sum1/1 -> Display6/1, Discrete-Time Integrator1/1
  Sum/1 -> Display5/1, Discrete-Time Integrator/1
  Discrete-Time Integrator1/1 -> y/1
  Bus Selector/3 -> Display1/1, Deadband1/1  "<y>"
  Bus Selector/5 -> mode/1  "<mode_switch>"
  Gain/1 -> Display7/1, <z>/1
  Deadband3/1 -> Gain/1  "z"

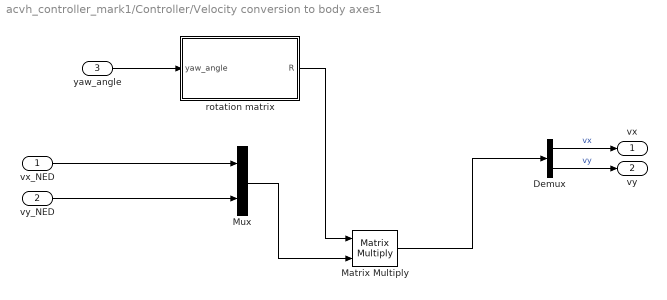
== system acvh_controller_mark1/Controller/Velocity conversion to body axes1 ==
  vx_NED : Inport
  vy_NED : Inport  Port=2
  yaw_angle : Inport  Port=3
  Demux : Demux  Outputs=2
  Matrix Multiply : Product  Multiplication=Matrix(*)
  Mux : Mux  Inputs=2
  rotation matrix : Subsystem
  vx : Outport
  vy : Outport  Port=2
  wires:
  vy_NED/1 -> Mux/2
  vx_NED/1 -> Mux/1
  Demux/1 -> vx/1  "vx"
  Demux/2 -> vy/1  "vy"
  rotation matrix/1(R) -> Matrix Multiply/1
  Matrix Multiply/1 -> Demux/1
  yaw_angle/1 -> rotation matrix/1(yaw_angle)
  Mux/1 -> Matrix Multiply/2

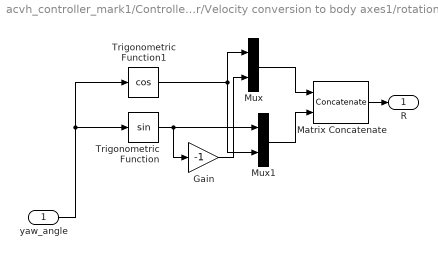
== system acvh_controller_mark1/Controller/Velocity conversion to body axes1/rotation matrix ==
  yaw_angle : Inport
  Gain : Gain  Gain=-1
  Matrix Concatenate : Concatenate  Mode=Multidimensional array  ConcatenateDimension=2
  Mux : Mux  Inputs=2
  Mux1 : Mux  Inputs=2
  Trigonometric Function : Trigonometry
  Trigonometric Function1 : Trigonometry  Operator=cos
  R : Outport
  wires:
  Mux1/1 -> Matrix Concatenate/2
  Trigonometric Function1/1 -> Mux1/2, Mux/1
  yaw_angle/1 -> Trigonometric Function1/1, Trigonometric Function/1
  Trigonometric Function/1 -> Gain/1, Mux1/1
  Mux/1 -> Matrix Concatenate/1
  Gain/1 -> Mux/2
  Matrix Concatenate/1 -> R/1

== matlab function acvh_controller_mark1/Controller/MATLAB Function1 ==
  data: des_vx input; tau_roll output; des_vy input; tau_pitch output; r input; p input
function [tau_roll, tau_pitch] = fcn(des_vx, des_vy, r, p)
    
    if(des_vx == 0)
        tau_pitch = 0;
    else
        tau_pitch = p;
    end
    if(des_vy == 0)
        tau_roll = 0;
    else
        tau_roll = r;
    end
end
